simulink model "kdt2simulatsioon"  (R2020b)
settings: Solver=VariableStepAuto  StartTime=0.0  StopTime=40  RelTol=1e-3
values from neighbouring files (symbols this model uses):
  A = [2.2 4.3 ... (first row only)    [YL_D_12.m]    (also in YL_E_9.m = [0.3479 0.6521 0.6521 0.3479]; analuus.m = [1 0;2 -2], B=[-2; -1], K=[0 0]; kodutoo1.m = [ 0 0 1 0;  0 0 0 1;  0 m*g/M -D/M 0;  0 -(M+m)*g/(M*L) D/(M)
  B = [0; 0; 1/M; -1/(M*L)]    [kodutoo1.m]    (also in lorentz.m = [0.,0.,0.1])
  C = 0.47    [hansuhw.m]    (also in kodutoo1.m = [1 L 0 0])
  G = [0; 0; 0; -1/(m*L)]    [kodutoo1.m]
  K = place(A, B, [P; -wn; -wn*1.2])    [kasufail.m]    (also in kodutoo2kasufail.m)
  K2d = dlqr(A2d,B2d,Q2d,R)    [kodutoo2kasufail.m]
  td = 0.2    [kasufail.m]    (also in kodutoo2kasufail.m)
  X1s = (9.5-0.5*nr)    [kodutoo1.m]
undefined symbols (not defined in the file or in its folder): Ad, Bd, Gd
settings Model: Creator=risto  LastModifiedBy=risto

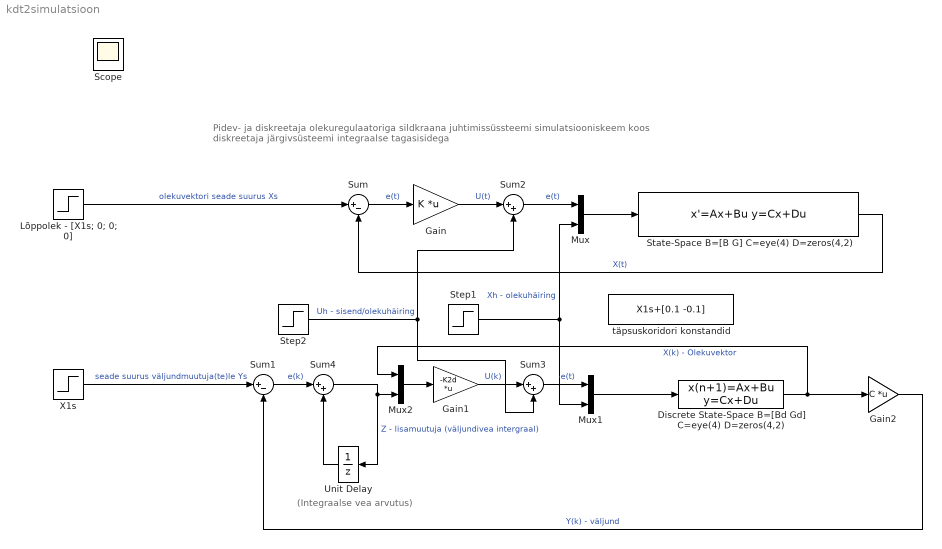
== system kdt2simulatsioon ==
  note: Pidev- ja diskreetaja olekuregulaatoriga sildkraana juhtimissüssteemi simulatsiooniskeem koos diskreetaja järgivsüsteemi integraalse tagasisidega
  note: (Integraalse vea arvutus)
  " X1s" : Step  Time=0  After=X1s  SampleTime=0
  Discrete State-Space B=[Bd Gd] C=eye(4) D=zeros(4,2) : DiscreteStateSpace  A=Ad  B=[Bd Gd]  C=eye(4)  D=zeros(4,2)  SampleTime=td
  Gain : Gain  Gain=K  Multiplication=Matrix(K*u)
  Gain1 : Gain  Gain=-K2d  Multiplication=Matrix(K*u)
  Gain2 : Gain  Gain=C  Multiplication=Matrix(K*u)
  Lõppolek - [X1s; 0; 0; 0] : Step  Time=0  After=[X1s; 0; 0; 0]  SampleTime=0
  Mux : Mux  Inputs=2
  Mux1 : Mux  Inputs=2
  Mux2 : Mux  Inputs=2
  State-Space B=[B G] C=eye(4) D=zeros(4,2) : StateSpace  A=A  B=[B G]  C=eye(4)  D=zeros(4,2)  InitialCondition=0
  Step1 : Step  Time=17  After=0  SampleTime=0
  Step2 : Step  Time=17  After=155  SampleTime=0
  Sum : Sum  Inputs=|+-
  Sum1 : Sum  Inputs=|+-
  Sum2 : Sum  Inputs=|++
  Sum3 : Sum  Inputs=|++
  Sum4 : Sum  Inputs=|++
  Unit Delay : UnitDelay  SampleTime=td  HasFrameUpgradeWarning=on
  täpsuskoridori konstandid : Constant  Value=X1s+[0.1 -0.1]
  Scope : Scope
  wires:
  Sum/1 -> Gain/1  "e(t)"
  Gain/1 -> Sum2/1  "U(t)"
  Mux/1 -> State-Space B=[B G] C=eye(4) D=zeros(4,2)/1
  State-Space B=[B G] C=eye(4) D=zeros(4,2)/1 -> Sum/2  "X(t)"
  Step1/1 -> Mux1/2, Mux/2  "Xh - olekuhäiring"
  Discrete State-Space B=[Bd Gd] C=eye(4) D=zeros(4,2)/1 -> Gain2/1, Mux2/1  "X(k) - Olekuvektor"
  Mux1/1 -> Discrete State-Space B=[Bd Gd] C=eye(4) D=zeros(4,2)/1
  Lõppolek - [X1s; 0; 0; 0]/1 -> Sum/1  "olekuvektori seade suurus Xs"
  Sum2/1 -> Mux/1  "e(t)"
  Step2/1 -> Sum2/2, Sum3/2  "Uh - sisend/olekuhäiring"
  Gain1/1 -> Sum3/1  "U(k)"
  Sum3/1 -> Mux1/1  "e(t)"
  Mux2/1 -> Gain1/1
  " X1s"/1 -> Sum1/1  "seade suurus väljundmuutuja(te)le Ys"
  Sum1/1 -> Sum4/1  "e(k)"
  Sum4/1 -> Unit Delay/1, Mux2/2  "Z - lisamuutuja (väljundivea intergraal)"
  Unit Delay/1 -> Sum4/2
  Gain2/1 -> Sum1/2  "Y(k) - väljund"
